simulink model "New_Model_vmaRHTS_R2019b_2"  (R2023b)
settings: Solver=ode4  StartTime=0.0  StopTime=tend  FixedStep=dt  RelTol=1e-3
values from neighbouring files (symbols this model uses):
  Ag = zeros(15,1)    [New_Full.m]
  AgN = zeros(15,1)    [New_Ns1.m]    (also in New_Ns2.m)
  AgP = zeros(6,1)    [New_Ps.m]    (also in New_Ps1.m; New_Ps2.m)
  CNrt = CRrt    [New_Ns1.m]    (also in New_Ns2.m)
  CPrt = CRrt(locate2,locate2)    [New_Ps.m]    (also in New_Ps1.m = alphas(1) * MPrt + alphas(2) * KPrt; New_Ps2.m = alphas(1) * MPrt + alphas(2) * KPrt)
  CRrt = alphas(1) * MRrt + alphas(2) * KRrt    [New_Full.m]
  dt = 1/1024    (= 0.0009765625)    [New_Full.m]
  FN = zeros(15,1)    [New_Full.m]    (also in New_Ns1.m; New_Ns2.m)
  K_P1 = zeros(6,5)    [New_Guyan.m]
  K_P2 = zeros(6,1)    [New_Guyan.m]
  Kbar_inv = inv(Kbar)    [New_Full.m]
  KNbar_inv = inv(KNbar)    [New_Ns1.m]    (also in New_Ns2.m)
  KPbar_inv = inv(KPbar)    [New_Ps.m]    (also in New_Ps1.m; New_Ps2.m)
  KPrt = KRrt(locate2,locate2)    [New_Ps.m]    (also in New_Ps1.m = [2*Kc(4,4)+2*Kc(1,1)	Kc(4,6)+Kc(1,3)	Kc(4,6)+Kc(1,3); New_Ps2.m = [2*Kc(4,4)+2*Kc(1,1)	Kc(4,6)+Kc(1,3)	Kc(4,6)+Kc(1,3)	2*Kc(1,)
  KPuc = KPrt(locate5,locate4)    [New_Guyan.m]
  KPuu = KPrt(locate5,locate5)    [New_Guyan.m]
  KRrt = [4*Kc(4,4)+4*Kc(1,1)	Kc(4,6)+Kc(1,3)	Kc(4,6)+Kc(1,3)	Kc(4,6)+Kc(1,3)	Kc(4,6)+Kc(1,3)	4*Kc(1,4)	Kc(1,6)	Kc(1,6)	Kc(1,6)	Kc(1,6)	0	0	0	0	0 ... (first row only)    [New_Full.m]
  l = zeros(15,1)    [New_Full.m]
  lN = zeros(15,1)    [New_Ns1.m]    (also in New_Ns2.m)
  locate2 = [1,2,3]    [New_Ns1.m]    (also in New_Ns2.m = [1,2,3,6,7,8]; New_Ps.m = [1,2,3,6,7,8]; New_Ps1.m = [1,2,3,6,7,8]; New_Ps2.m = [1,2,3,6,7,8])
  locate3 = zeros(15,6)    [New_Ns1.m]    (also in New_Ns2.m)
  lP = zeros(6,1)    [New_Ps.m]    (also in New_Ps1.m; New_Ps2.m)
  MNrt = diag([M5 1e-5 M6 M3 M2 M1 M2 M3 M3 M2 M1 M2 M3 M3 M2])    [New_Ns1.m]    (also in New_Ns2.m = diag([M5 1e-5 M6 M3 M2 M5 1e-5 M6 M3 M2 M1 M2 M3 M3 M2]))
  MPrt = diag([M4 M2 M3 M4 M2 M3])    [New_Ps.m]    (also in New_Ps1.m = diag([M4 M2 M2]); New_Ps2.m = diag([M4 M2 M2 M4 M2 M2]))
  MPuu = MPrt(locate5,locate5)    [New_Guyan.m]
  MRrt = diag([M1 M2 M3 M3 M2 M1 M2 M3 M3 M2 M1 M2 M3 M3 M2])    [New_Full.m]
  Rbar = zeros(15,1)    [New_Full.m]
  RNbar = zeros(15,1)    [New_Ns1.m]    (also in New_Ns2.m)
  RPbar = zeros(6,1)    [New_Ps.m]    (also in New_Ps1.m; New_Ps2.m)
  tend = 40    [New_Full.m]
undefined symbols (not defined in the file or in its folder): a0, a1, a2, a3, a4, a5, a6, a7, Ag_tilde, C_tilde, Cp_tilde, CPren, Cren, EQ_intensity, EQ_sw, F_tilde, Klocate1, KN_tilde_inv, KNren_inv, Koo, Kot, Kp_tilde, KPren, Ksmn, Ksn, l_tilde, lren, M_tilde, Mp_tilde, MPren, Mren, Phi_u0, R_tilde, Rren, T
libraries: simulink x1, sldrtlib x1
(part 1 of 2)
settings Model: Creator=icu327  LastModifiedBy=liangyu
settings DataIOCC: SaveFormat=Array  ReturnWorkspaceOutputs=off
settings DebuggingCC: UnconnectedInputMsg=warning  UnconnectedOutputMsg=warning  UnconnectedLineMsg=warning  ArithmeticOperatorsInVariantConditions=warning
settings HardwareCC: ProdBitPerLong=64  ProdHWDeviceType=Intel->x86-64 (Linux 64)
settings ModelReferenceCC: EnableRefExpFcnMdlSchedulingChecks=on
settings SFSimCC: CustomCodeUndefinedFunction=UseInterfaceOnly
settings RTWCC: Description=Simulink Desktop Real-Time  SystemTargetFile=sldrt.tlc  TemplateMakefile=sldrt.tmf  RTWCompilerOptimization=on
settings CodeAppCC: MaxIdLength=95  StateflowObjectComments=on
settings SimulinkDesktopRealTimeCC: TargetLibSuffix=_sldrt.a  TargetPreCompLibLocation=C:\Program Files\MATLAB\R2023b\toolbox\sldrt\lib\win64

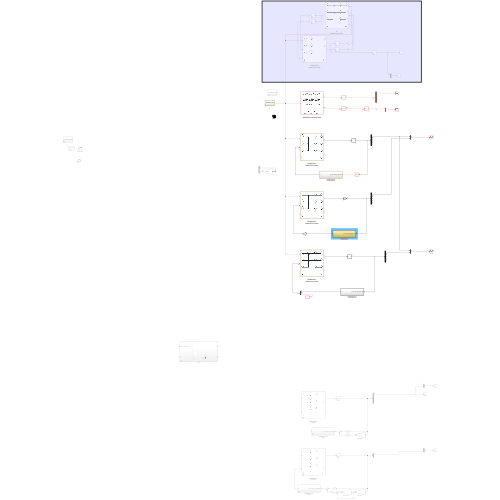
[thumbnail: Simulink's stored preview of the top-level diagram]
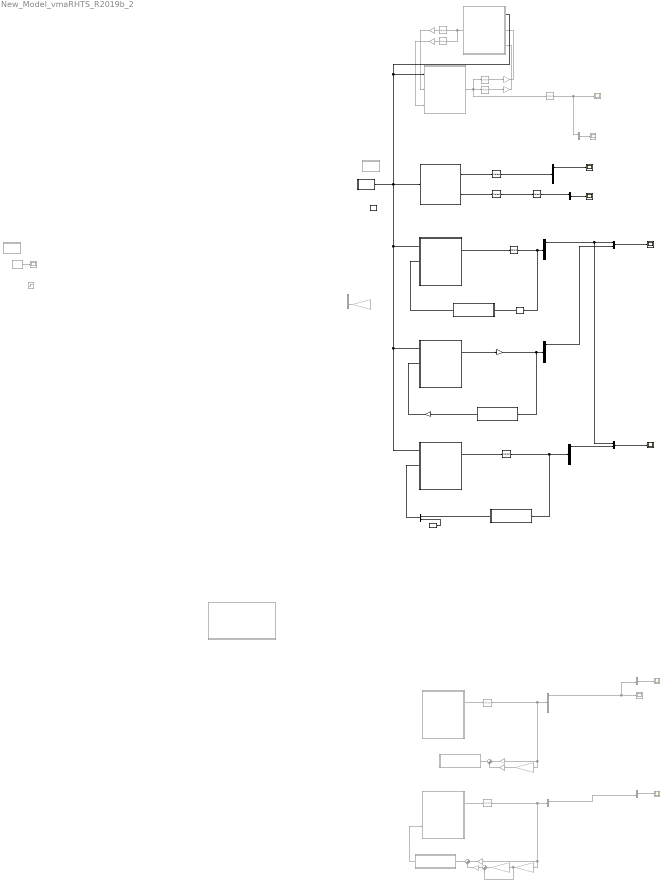
== system New_Model_vmaRHTS_R2019b_2 ==
  " 1" : Subsystem  Commented=on
  " 2" : Subsystem
  " 3" : Subsystem  Commented=on
  " NUMERICAL Guyan" : Subsystem  Commented=on
      mask Display: image('$imagefile'); % Use "Edit Image" on toolstrip to change.
  " NUMERICAL Guyan1" : Subsystem  Commented=on
      mask Display: image('$imagefile'); % Use "Edit Image" on toolstrip to change.
  " NUMERICAL SUBSTRUCTURE" : Subsystem  Commented=on
      mask Display: image('$imagefile'); % Use "Edit Image" on toolstrip to change.
  " NUMERICAL SUBSTRUCTURE1" : Subsystem
      mask Display: image('$imagefile'); % Use "Edit Image" on toolstrip to change.
  " NUMERICAL SUBSTRUCTURE2" : Subsystem
      mask Display: image('$imagefile'); % Use "Edit Image" on toolstrip to change.
  " NUMERICAL SUBSTRUCTURE3" : Subsystem
      mask Display: image('$imagefile'); % Use "Edit Image" on toolstrip to change.
  " Ps SUBSTRUCTURE1" : Subsystem  Commented=on
      mask Display: image('$imagefile'); % Use "Edit Image" on toolstrip to change.
  " REFERENCE STRUCTURE" : Subsystem
      mask Display: image('$imagefile'); % Use "Edit Image" on toolstrip to change.
  CBtest : Subsystem  Commented=on
  Chirp Signal1 : simulink/Sources/Chirp Signal  f1=0.1  T=tend  f2=10
  Constant3 : Constant  Value=zeros(3,1)  VectorParams1D=off
  Delay : Delay
  Demux : Demux  Outputs=6
  Demux1 : Demux  Outputs=6
  Demux2 : Demux  Commented=on  Outputs=5
  Demux3 : Demux  Commented=on  Outputs=2
  Demux4 : Demux  Outputs=5
  Demux5 : Demux  Outputs=5
  Feedback Force Computation1 : Subsystem
  Feedback Force Computation2 : Subsystem
  Feedback Force Computation3 : Subsystem
  Feedback Force Guyan : Subsystem  Commented=on
  Feedback Force Guyan1 : Subsystem  Commented=on
  Gain : Gain  Commented=on  Gain=K_P1  Multiplication=Matrix(K*u) (u vector)
  Gain1 : Gain  Commented=on  Gain=KRrt(3,4)  Multiplication=Matrix(K*u) (u vector)
  Gain11 : Gain  Commented=on  Gain=-inv(Koo)*Kot  Multiplication=Matrix(K*u) (u vector)
  Gain2 : Gain  Commented=on  Gain=KRrt(7:8,9:13)  Multiplication=Matrix(K*u) (u vector)
  Gain3 : Gain  Commented=on  Gain=KRrt(4,3)  Multiplication=Matrix(K*u) (u vector)
  Gain4 : Gain  Commented=on  Gain=KRrt(9:13,7:8)  Multiplication=Matrix(K*u) (u vector)
  Gain5 : Gain  Commented=on  Gain=K_P2  Multiplication=Matrix(K*u) (u vector)
  Gain6 : Gain  Commented=on  Gain=K_P1  Multiplication=Matrix(K*u) (u vector)
  Gain7 : Gain  Commented=on  Gain=K_P2  Multiplication=Matrix(K*u) (u vector)
  Gain8 : Gain  Gain=Klocate1  Multiplication=Matrix(K*u) (u vector)
  Gain9 : Gain  Gain=Klocate1'  Multiplication=Matrix(K*u) (u vector)
  Guyan增益 : Gain  Commented=on  Gain=-inv(KPuu)*KPuc  Multiplication=Matrix(K*u) (u vector)
  Guyan增益1 : Gain  Commented=on  Gain=-inv(KPuu)*KPuc  Multiplication=Matrix(K*u) (u vector)
  Guyan增益2 : Gain  Commented=on  Gain=Phi_u0*Phi_u0' * MPuu  Multiplication=Matrix(K*u) (u vector)
  Missed Ticks : Scope  Commented=on
  Mux{,6,8..9} (4 alike) : Mux  Commented=on  Inputs=2
  Mux{1..3,5} (4 alike) : Mux  Inputs=2
  Real-Time Synchronization : sldrtlib/Real-Time Synchronization  Commented=on  SampleTime=dt  MaxMissedTicks=10000  ShowMissedTicks=on  YieldWhenWaiting=off
  Scope{,3..5} (4 alike) : Scope
  Scope{1..2,11..13} (5 alike) : Scope  Commented=on
  Selector : Selector  InputPortWidth=15  IndexOptions=Index vector (dialog)  Indices=[1 2 3 6 7 8]  OutputSizes=1
  Selector1 : Selector  Commented=on  InputPortWidth=11  IndexOptions=Index vector (dialog)  Indices=[2]  OutputSizes=1
  Selector11 : Selector  InputPortWidth=6  IndexOptions=Index vector (dialog)  Indices=[1]  OutputSizes=1
  Selector12 : Selector  InputPortWidth=15  IndexOptions=Index vector (dialog)  Indices=[1 2 3 6 7 8]  OutputSizes=1
  Selector13 : Selector  Commented=on  InputPortWidth=15  IndexOptions=Index vector (dialog)  Indices=[1 3 6 7 8]  OutputSizes=1
  Selector2 : Selector  Commented=on  InputPortWidth=11  IndexOptions=Index vector (dialog)  Indices=[5 6 7 8 9]  OutputSizes=1
  Selector3 : Selector  Commented=on  InputPortWidth=15  IndexOptions=Index vector (dialog)  Indices=[1 3 6 7 8]  OutputSizes=1
  Selector4 : Selector  Commented=on  InputPortWidth=11  IndexOptions=Index vector (dialog)  Indices=[1]  OutputSizes=1
  Selector5 : Selector  InputPortWidth=15  IndexOptions=Index vector (dialog)  Indices=[1 2 3 6 7 8]  OutputSizes=1
  Selector6 : Selector  Commented=on  InputPortWidth=6  IndexOptions=Index vector (dialog)  Indices=[3]  OutputSizes=1
  Selector7 : Selector  Commented=on  InputPortWidth=6  IndexOptions=Index vector (dialog)  Indices=[5 6]  OutputSizes=1
  Selector8 : Selector  InputPortWidth=8  IndexOptions=Index vector (dialog)  Indices=[1 2 3 4 5]  OutputSizes=1
  Step5 : Step  Commented=on  SampleTime=0
  Sum : Sum  Commented=on  Inputs=|++
  Sum2 : Sum  Commented=on  Inputs=|++
  Sum3 : Sum  Commented=on  Inputs=|++
  wires:
  Real-Time Synchronization/1 -> Missed Ticks/1
  " REFERENCE STRUCTURE"/1(Output) -> Selector5/1
  Mux/1 -> Scope2/1
  " Ps SUBSTRUCTURE1"/1(Output) -> Selector7/1, Selector6/1
  Selector4/1 -> Scope1/1, Mux/1
  Selector2/1 -> Gain2/1
  Selector1/1 -> Gain1/1
  Gain1/1 -> " Ps SUBSTRUCTURE1"/2(Input)
  Gain2/1 -> " Ps SUBSTRUCTURE1"/3(Input1)
  Selector6/1 -> Gain3/1
  Gain3/1 -> " NUMERICAL SUBSTRUCTURE"/2(Input)
  Selector7/1 -> Gain4/1
  Gain4/1 -> " NUMERICAL SUBSTRUCTURE"/3(Input1)
  " NUMERICAL SUBSTRUCTURE"/1(Output) -> Selector4/1, Selector1/1, Selector2/1
  Selector12/1 -> Selector11/1
  " REFERENCE STRUCTURE"/2(Output1) -> Selector12/1
  Selector11/1 -> Mux1/1  "Rs"
  Mux1/1 -> Scope3/1
  Selector5/1 -> Demux1/1  "Rs"
  Demux1/1 -> Scope4/1
  " NUMERICAL Guyan"/1(Output) -> Selector3/1
  Guyan增益/1 -> Gain5/1
  Sum/1 -> Feedback Force Guyan/1("[x_est, theta_est] (m,rad)")
  Gain/1 -> Sum/1
  Gain5/1 -> Sum/2
  Demux2/1 -> Scope11/1, Mux8/2  "Ns"
  Mux8/1 -> Scope12/1
  Gain6/1 -> Sum2/1
  Feedback Force Guyan1/1(Output) -> " NUMERICAL Guyan1"/2(Input)
  Guyan增益1/1 -> Guyan增益2/1, Sum3/2
  Sum2/1 -> Feedback Force Guyan1/1("[x_est, theta_est] (m,rad)")
  " NUMERICAL Guyan1"/1(Output) -> Selector13/1
  Gain7/1 -> Sum2/2
  Guyan增益2/1 -> Sum3/1
  Sum3/1 -> Gain7/1
  Demux3/1 -> Mux9/2  "Ns"
  Mux9/1 -> Scope13/1
  Selector3/1 -> Demux2/1, Guyan增益/1, Gain/1
  Selector13/1 -> Demux3/1, Guyan增益1/1, Gain6/1
  Feedback Force Computation3/1(Output) -> " NUMERICAL SUBSTRUCTURE1"/2(Input)
  Gain9/1 -> " NUMERICAL SUBSTRUCTURE2"/2(Input)
  Demux4/1 -> Mux2/2  "Ns"
  ? -> Gain11/1
  ? -> Mux6/1
  Gain11/1 -> Mux6/2
  Gain8/1 -> Feedback Force Computation1/1("[x_est, theta_est] (m,rad)"), Demux4/1
  " NUMERICAL SUBSTRUCTURE3"/1(Output) -> Selector8/1
  " 2"/1(GROUND ACCEL) -> " NUMERICAL SUBSTRUCTURE2"/1(Ground_Acceleration), " NUMERICAL SUBSTRUCTURE3"/1(Ground_Acceleration), " NUMERICAL SUBSTRUCTURE1"/1(Ground_Acceleration), " NUMERICAL SUBSTRUCTURE"/1(Ground_Acceleration), " Ps SUBSTRUCTURE1"/1(Ground_Acceleration), " REFERENCE STRUCTURE"/1(Ground_Acceleration)
  Mux5/1 -> " NUMERICAL SUBSTRUCTURE3"/2(Input)
  Constant3/1 -> Mux5/2
  Selector8/1 -> Feedback Force Computation2/1("[x_est, theta_est] (m,rad)"), Demux5/1
  Feedback Force Computation2/1(Output) -> Mux5/1
  Feedback Force Computation1/1(Output) -> Gain9/1
  " NUMERICAL SUBSTRUCTURE2"/1(Output) -> Gain8/1
  " NUMERICAL SUBSTRUCTURE1"/1(Output) -> Selector/1
  Demux/1 -> Mux3/1, Mux2/1  "Ns"
  Mux2/1 -> Scope/1
  Mux3/1 -> Scope5/1
  Demux5/1 -> Mux3/2  "Ns"
  Selector/1 -> Delay/1, Demux/1
  Delay/1 -> Feedback Force Computation3/1("[x_est, theta_est] (m,rad)")

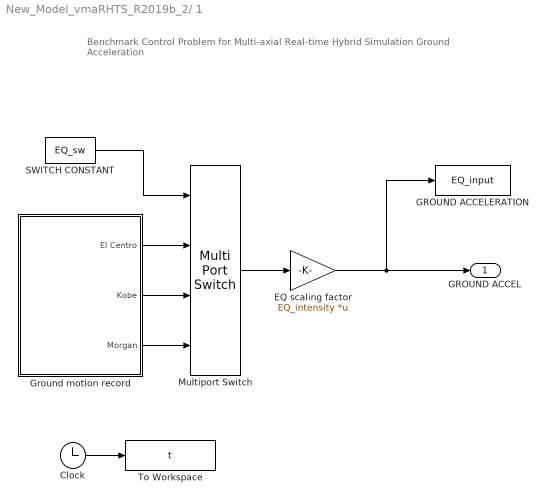
== system New_Model_vmaRHTS_R2019b_2/ 1 ==
  note: Benchmark Control Problem for
      | Multi-axial Real-time Hybrid Simulation
      | Ground Acceleration
  Clock : Clock
  EQ scaling factor : Gain  Gain=EQ_intensity  Multiplication=Matrix(K*u)
  GROUND ACCELERATION : ToWorkspace  VariableName=EQ_input  SampleTime=-1
      settings: Save2DSignal=2-D array (concatenate along first dimension)
  Ground motion record : Subsystem
  Multiport Switch : MultiPortSwitch  SaturateOnIntegerOverflow=off  InputSameDT=off
  SWITCH CONSTANT : Constant  Value=EQ_sw
  To Workspace : ToWorkspace  VariableName=t  SampleTime=dt
  GROUND ACCEL : Outport  VectorParamsAs1DForOutWhenUnconnected=off
  wires:
  Multiport Switch/1 -> EQ scaling factor/1
  EQ scaling factor/1 -> GROUND ACCELERATION/1, GROUND ACCEL/1
  Ground motion record/1(El Centro) -> Multiport Switch/2
  Ground motion record/2(Kobe) -> Multiport Switch/3
  Ground motion record/3(Morgan) -> Multiport Switch/4
  SWITCH CONSTANT/1 -> Multiport Switch/1
  Clock/1 -> To Workspace/1

== system New_Model_vmaRHTS_R2019b_2/ 2 ==
  note: Benchmark Control Problem for
      | Multi-axial Real-time Hybrid Simulation
      | Ground Acceleration
  Clock : Clock
  EQ scaling factor : Gain  Gain=EQ_intensity  Multiplication=Matrix(K*u)
  GROUND ACCELERATION : ToWorkspace  VariableName=EQ_input  SampleTime=-1
      settings: Save2DSignal=2-D array (concatenate along first dimension)
  Ground motion record : Subsystem
  Multiport Switch : MultiPortSwitch  SaturateOnIntegerOverflow=off  InputSameDT=off
  SWITCH CONSTANT : Constant  Value=EQ_sw
  To Workspace : ToWorkspace  VariableName=t  SampleTime=dt
  GROUND ACCEL : Outport  VectorParamsAs1DForOutWhenUnconnected=off
  wires:
  Multiport Switch/1 -> EQ scaling factor/1
  EQ scaling factor/1 -> GROUND ACCELERATION/1, GROUND ACCEL/1
  Ground motion record/1(El Centro) -> Multiport Switch/2
  Ground motion record/2(Kobe) -> Multiport Switch/3
  Ground motion record/3(Morgan) -> Multiport Switch/4
  SWITCH CONSTANT/1 -> Multiport Switch/1
  Clock/1 -> To Workspace/1

== system New_Model_vmaRHTS_R2019b_2/ 3 ==
  note: Benchmark Control Problem for
      | Multi-axial Real-time Hybrid Simulation
      | Ground Acceleration
  Clock : Clock
  EQ scaling factor : Gain  Gain=EQ_intensity  Multiplication=Matrix(K*u)
  GROUND ACCELERATION : ToWorkspace  VariableName=EQ_input  SampleTime=-1
      settings: Save2DSignal=2-D array (concatenate along first dimension)
  Ground motion record : Subsystem
  Multiport Switch : MultiPortSwitch  SaturateOnIntegerOverflow=off  InputSameDT=off
  SWITCH CONSTANT : Constant  Value=EQ_sw
  To Workspace : ToWorkspace  VariableName=t  SampleTime=dt
  GROUND ACCEL : Outport  VectorParamsAs1DForOutWhenUnconnected=off
  wires:
  Multiport Switch/1 -> EQ scaling factor/1
  EQ scaling factor/1 -> GROUND ACCELERATION/1, GROUND ACCEL/1
  Ground motion record/1(El Centro) -> Multiport Switch/2
  Ground motion record/2(Kobe) -> Multiport Switch/3
  Ground motion record/3(Morgan) -> Multiport Switch/4
  SWITCH CONSTANT/1 -> Multiport Switch/1
  Clock/1 -> To Workspace/1

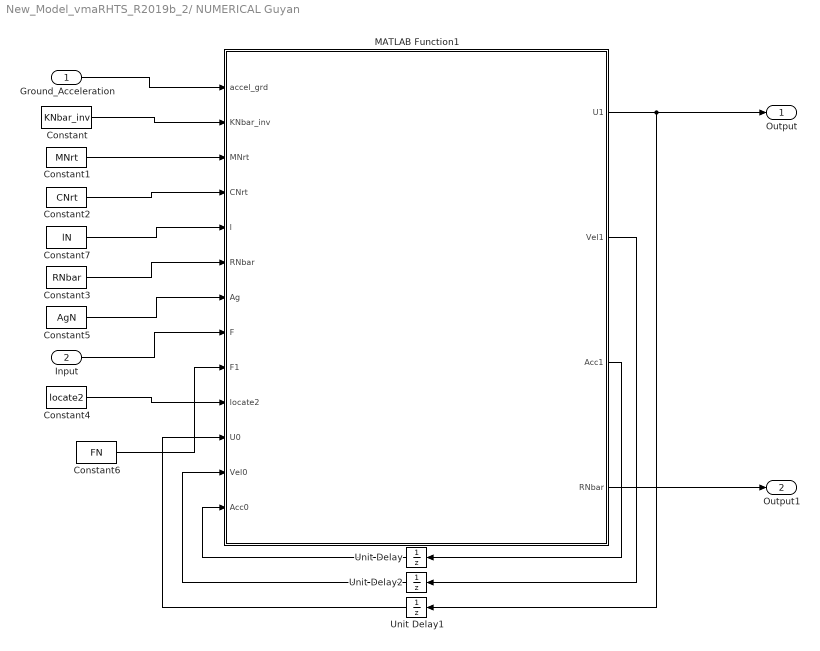
== system New_Model_vmaRHTS_R2019b_2/ NUMERICAL Guyan ==
  Ground_Acceleration : Inport
  Input : Inport  Port=2
  Constant : Constant  Value=KNbar_inv  VectorParams1D=off
  Constant1 : Constant  Value=MNrt  VectorParams1D=off
  Constant2 : Constant  Value=CNrt  VectorParams1D=off
  Constant3 : Constant  Value=RNbar  VectorParams1D=off
  Constant4 : Constant  Value=locate2  VectorParams1D=off
  Constant5 : Constant  Value=AgN  VectorParams1D=off
  Constant6 : Constant  Value=FN  VectorParams1D=off
  Constant7 : Constant  Value=lN  VectorParams1D=off
  MATLAB Function1 : MATLAB Function  TreatAsAtomicUnit=on
  Unit Delay : UnitDelay  SampleTime=-1  HasFrameUpgradeWarning=on
  Unit Delay1 : UnitDelay  SampleTime=-1  HasFrameUpgradeWarning=on
  Unit Delay2 : UnitDelay  SampleTime=-1  HasFrameUpgradeWarning=on
  Output : Outport
  Output1 : Outport  Port=2
  wires:
  Ground_Acceleration/1 -> MATLAB Function1/1(accel_grd)
  Constant/1 -> MATLAB Function1/2(KNbar_inv)
  Constant1/1 -> MATLAB Function1/3(MNrt)
  Constant2/1 -> MATLAB Function1/4(CNrt)
  Constant7/1 -> MATLAB Function1/5(l)
  Unit Delay2/1 -> MATLAB Function1/12(Vel0)
  Unit Delay/1 -> MATLAB Function1/13(Acc0)
  MATLAB Function1/2(Vel1) -> Unit Delay2/1
  MATLAB Function1/3(Acc1) -> Unit Delay/1
  Constant5/1 -> MATLAB Function1/7(Ag)
  Unit Delay1/1 -> MATLAB Function1/11(U0)
  Constant3/1 -> MATLAB Function1/6("RNbar ")
  Input/1 -> MATLAB Function1/8(F)
  MATLAB Function1/1(U1) -> Output/1, Unit Delay1/1
  Constant4/1 -> MATLAB Function1/10(locate2)
  Constant6/1 -> MATLAB Function1/9(F1)
  MATLAB Function1/4(RNbar) -> Output1/1

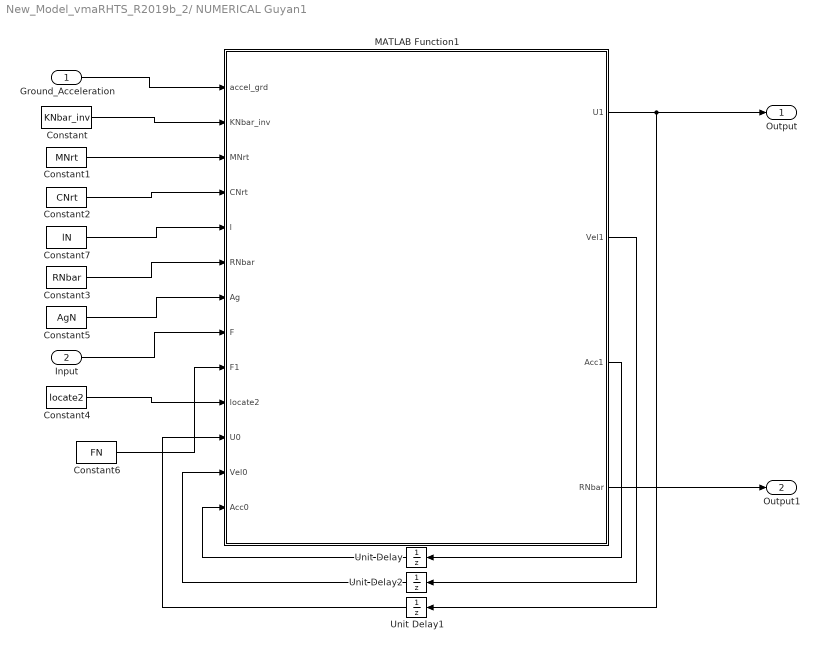
== system New_Model_vmaRHTS_R2019b_2/ NUMERICAL Guyan1 ==
  Ground_Acceleration : Inport
  Input : Inport  Port=2
  Constant : Constant  Value=KNbar_inv  VectorParams1D=off
  Constant1 : Constant  Value=MNrt  VectorParams1D=off
  Constant2 : Constant  Value=CNrt  VectorParams1D=off
  Constant3 : Constant  Value=RNbar  VectorParams1D=off
  Constant4 : Constant  Value=locate2  VectorParams1D=off
  Constant5 : Constant  Value=AgN  VectorParams1D=off
  Constant6 : Constant  Value=FN  VectorParams1D=off
  Constant7 : Constant  Value=lN  VectorParams1D=off
  MATLAB Function1 : MATLAB Function  TreatAsAtomicUnit=on
  Unit Delay : UnitDelay  SampleTime=-1  HasFrameUpgradeWarning=on
  Unit Delay1 : UnitDelay  SampleTime=-1  HasFrameUpgradeWarning=on
  Unit Delay2 : UnitDelay  SampleTime=-1  HasFrameUpgradeWarning=on
  Output : Outport
  Output1 : Outport  Port=2
  wires:
  Ground_Acceleration/1 -> MATLAB Function1/1(accel_grd)
  Constant/1 -> MATLAB Function1/2(KNbar_inv)
  Constant1/1 -> MATLAB Function1/3(MNrt)
  Constant2/1 -> MATLAB Function1/4(CNrt)
  Constant7/1 -> MATLAB Function1/5(l)
  Unit Delay2/1 -> MATLAB Function1/12(Vel0)
  Unit Delay/1 -> MATLAB Function1/13(Acc0)
  MATLAB Function1/2(Vel1) -> Unit Delay2/1
  MATLAB Function1/3(Acc1) -> Unit Delay/1
  Constant5/1 -> MATLAB Function1/7(Ag)
  Unit Delay1/1 -> MATLAB Function1/11(U0)
  Constant3/1 -> MATLAB Function1/6("RNbar ")
  Input/1 -> MATLAB Function1/8(F)
  MATLAB Function1/1(U1) -> Output/1, Unit Delay1/1
  Constant4/1 -> MATLAB Function1/10(locate2)
  Constant6/1 -> MATLAB Function1/9(F1)
  MATLAB Function1/4(RNbar) -> Output1/1

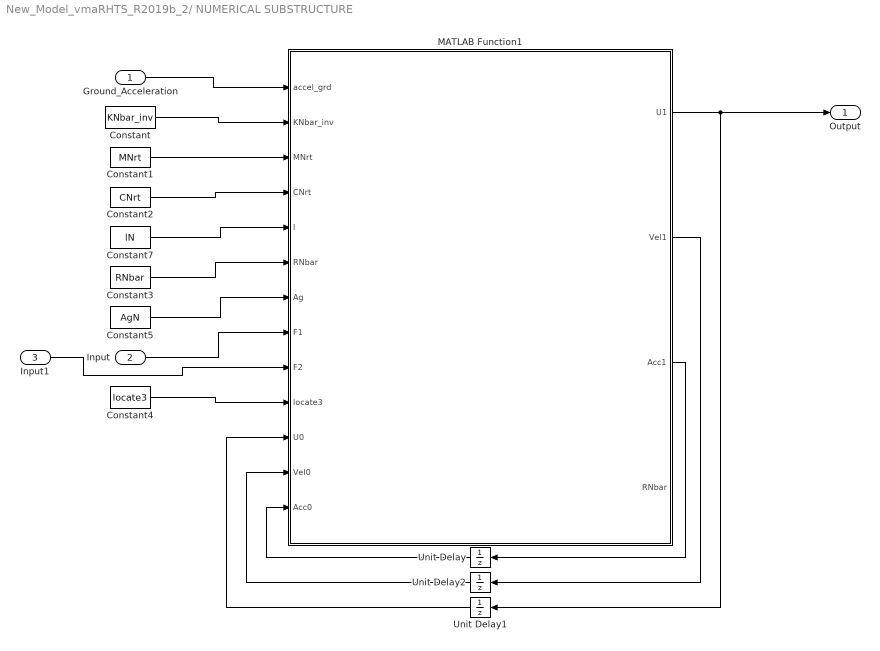
== system New_Model_vmaRHTS_R2019b_2/ NUMERICAL SUBSTRUCTURE ==
  Ground_Acceleration : Inport
  Input : Inport  Port=2
  Input1 : Inport  Port=3
  Constant : Constant  Value=KNbar_inv  VectorParams1D=off
  Constant1 : Constant  Value=MNrt  VectorParams1D=off
  Constant2 : Constant  Value=CNrt  VectorParams1D=off
  Constant3 : Constant  Value=RNbar  VectorParams1D=off
  Constant4 : Constant  Value=locate3  VectorParams1D=off
  Constant5 : Constant  Value=AgN  VectorParams1D=off
  Constant7 : Constant  Value=lN  VectorParams1D=off
  MATLAB Function1 : MATLAB Function  TreatAsAtomicUnit=on
  Unit Delay : UnitDelay  SampleTime=-1  HasFrameUpgradeWarning=on
  Unit Delay1 : UnitDelay  SampleTime=-1  HasFrameUpgradeWarning=on
  Unit Delay2 : UnitDelay  SampleTime=-1  HasFrameUpgradeWarning=on
  Output : Outport
  wires:
  Ground_Acceleration/1 -> MATLAB Function1/1(accel_grd)
  Constant/1 -> MATLAB Function1/2(KNbar_inv)
  Constant1/1 -> MATLAB Function1/3(MNrt)
  Constant2/1 -> MATLAB Function1/4(CNrt)
  Constant7/1 -> MATLAB Function1/5(l)
  Unit Delay2/1 -> MATLAB Function1/12(Vel0)
  Unit Delay/1 -> MATLAB Function1/13(Acc0)
  MATLAB Function1/2(Vel1) -> Unit Delay2/1
  MATLAB Function1/3(Acc1) -> Unit Delay/1
  Constant5/1 -> MATLAB Function1/7(Ag)
  Unit Delay1/1 -> MATLAB Function1/11(U0)
  Constant3/1 -> MATLAB Function1/6("RNbar ")
  Input/1 -> MATLAB Function1/8(F1)
  MATLAB Function1/1(U1) -> Output/1, Unit Delay1/1
  Constant4/1 -> MATLAB Function1/10(locate3)
  Input1/1 -> MATLAB Function1/9(F2)

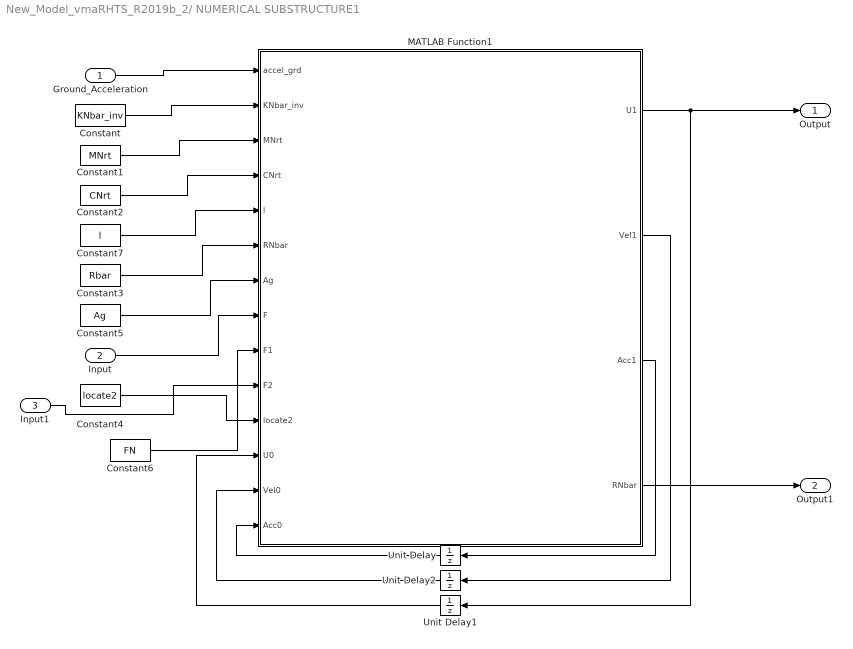
== system New_Model_vmaRHTS_R2019b_2/ NUMERICAL SUBSTRUCTURE1 ==
  Ground_Acceleration : Inport
  Input : Inport  Port=2
  Input1 : Inport  Port=3
  Constant : Constant  Value=KNbar_inv  VectorParams1D=off
  Constant1 : Constant  Value=MNrt  VectorParams1D=off
  Constant2 : Constant  Value=CNrt  VectorParams1D=off
  Constant3 : Constant  Value=Rbar  VectorParams1D=off
  Constant4 : Constant  Value=locate2  VectorParams1D=off
  Constant5 : Constant  Value=Ag  VectorParams1D=off
  Constant6 : Constant  Value=FN  VectorParams1D=off
  Constant7 : Constant  Value=l  VectorParams1D=off
  MATLAB Function1 : MATLAB Function  TreatAsAtomicUnit=on
  Unit Delay : UnitDelay  SampleTime=-1  HasFrameUpgradeWarning=on
  Unit Delay1 : UnitDelay  SampleTime=-1  HasFrameUpgradeWarning=on
  Unit Delay2 : UnitDelay  SampleTime=-1  HasFrameUpgradeWarning=on
  Output : Outport
  Output1 : Outport  Port=2
  wires:
  Ground_Acceleration/1 -> MATLAB Function1/1(accel_grd)
  Constant/1 -> MATLAB Function1/2(KNbar_inv)
  Constant1/1 -> MATLAB Function1/3(MNrt)
  Constant2/1 -> MATLAB Function1/4(CNrt)
  Constant7/1 -> MATLAB Function1/5(l)
  Unit Delay2/1 -> MATLAB Function1/13(Vel0)
  Unit Delay/1 -> MATLAB Function1/14(Acc0)
  MATLAB Function1/2(Vel1) -> Unit Delay2/1
  MATLAB Function1/3(Acc1) -> Unit Delay/1
  Constant5/1 -> MATLAB Function1/7(Ag)
  Unit Delay1/1 -> MATLAB Function1/12(U0)
  Constant3/1 -> MATLAB Function1/6("RNbar ")
  Input/1 -> MATLAB Function1/8(F)
  MATLAB Function1/1(U1) -> Output/1, Unit Delay1/1
  Constant4/1 -> MATLAB Function1/11(locate2)
  Constant6/1 -> MATLAB Function1/9(F1)
  MATLAB Function1/4(RNbar) -> Output1/1
  Input1/1 -> MATLAB Function1/10(F2)

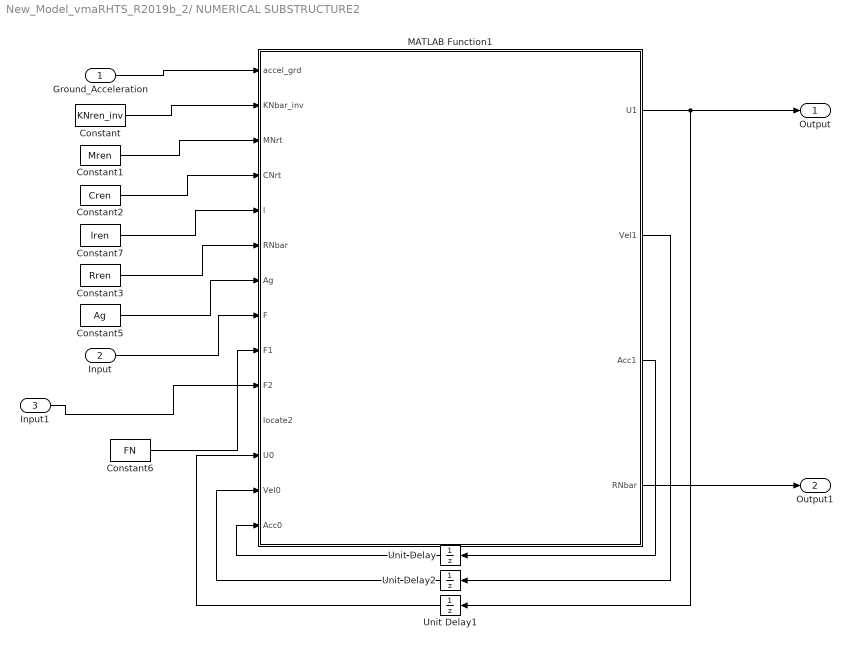
== system New_Model_vmaRHTS_R2019b_2/ NUMERICAL SUBSTRUCTURE2 ==
  Ground_Acceleration : Inport
  Input : Inport  Port=2
  Input1 : Inport  Port=3
  Constant : Constant  Value=KNren_inv  VectorParams1D=off
  Constant1 : Constant  Value=Mren  VectorParams1D=off
  Constant2 : Constant  Value=Cren  VectorParams1D=off
  Constant3 : Constant  Value=Rren  VectorParams1D=off
  Constant5 : Constant  Value=Ag  VectorParams1D=off
  Constant6 : Constant  Value=FN  VectorParams1D=off
  Constant7 : Constant  Value=lren  VectorParams1D=off
  MATLAB Function1 : MATLAB Function  TreatAsAtomicUnit=on
  Unit Delay : UnitDelay  SampleTime=-1  HasFrameUpgradeWarning=on
  Unit Delay1 : UnitDelay  SampleTime=-1  HasFrameUpgradeWarning=on
  Unit Delay2 : UnitDelay  SampleTime=-1  HasFrameUpgradeWarning=on
  Output : Outport
  Output1 : Outport  Port=2
  wires:
  Ground_Acceleration/1 -> MATLAB Function1/1(accel_grd)
  Constant/1 -> MATLAB Function1/2(KNbar_inv)
  Constant1/1 -> MATLAB Function1/3(MNrt)
  Constant2/1 -> MATLAB Function1/4(CNrt)
  Constant7/1 -> MATLAB Function1/5(l)
  Unit Delay2/1 -> MATLAB Function1/13(Vel0)
  Unit Delay/1 -> MATLAB Function1/14(Acc0)
  MATLAB Function1/2(Vel1) -> Unit Delay2/1
  MATLAB Function1/3(Acc1) -> Unit Delay/1
  Constant5/1 -> MATLAB Function1/7(Ag)
  Unit Delay1/1 -> MATLAB Function1/12(U0)
  Constant3/1 -> MATLAB Function1/6("RNbar ")
  Input/1 -> MATLAB Function1/8(F)
  MATLAB Function1/1(U1) -> Output/1, Unit Delay1/1
  Constant6/1 -> MATLAB Function1/9(F1)
  MATLAB Function1/4(RNbar) -> Output1/1
  Input1/1 -> MATLAB Function1/10(F2)

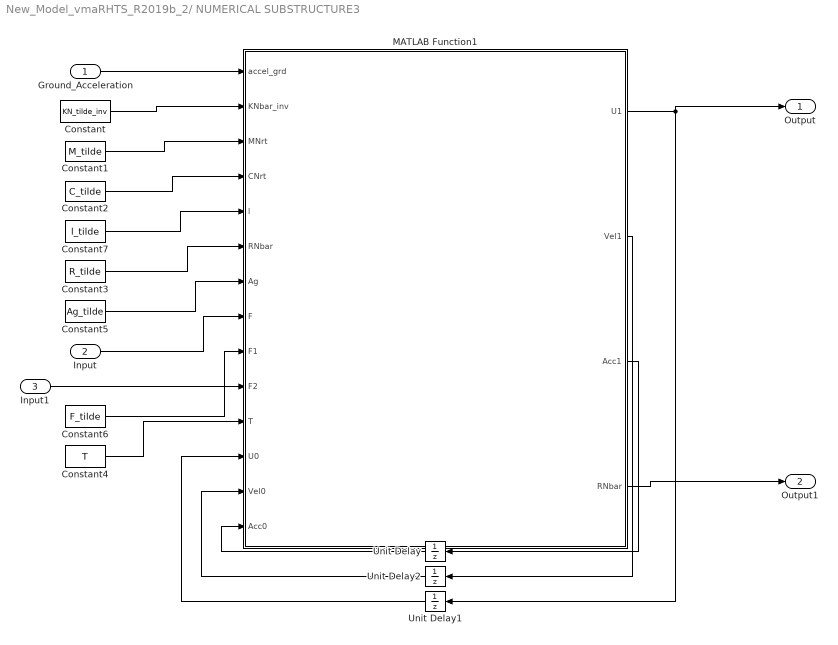
== system New_Model_vmaRHTS_R2019b_2/ NUMERICAL SUBSTRUCTURE3 ==
  Ground_Acceleration : Inport
  Input : Inport  Port=2
  Input1 : Inport  Port=3
  Constant : Constant  Value=KN_tilde_inv  VectorParams1D=off
  Constant1 : Constant  Value=M_tilde  VectorParams1D=off
  Constant2 : Constant  Value=C_tilde  VectorParams1D=off
  Constant3 : Constant  Value=R_tilde  VectorParams1D=off
  Constant4 : Constant  Value=T  VectorParams1D=off
  Constant5 : Constant  Value=Ag_tilde  VectorParams1D=off
  Constant6 : Constant  Value=F_tilde  VectorParams1D=off
  Constant7 : Constant  Value=l_tilde  VectorParams1D=off
  MATLAB Function1 : MATLAB Function  TreatAsAtomicUnit=on
  Unit Delay : UnitDelay  SampleTime=-1  HasFrameUpgradeWarning=on
  Unit Delay1 : UnitDelay  SampleTime=-1  HasFrameUpgradeWarning=on
  Unit Delay2 : UnitDelay  SampleTime=-1  HasFrameUpgradeWarning=on
  Output : Outport
  Output1 : Outport  Port=2
  wires:
  Ground_Acceleration/1 -> MATLAB Function1/1(accel_grd)
  Constant/1 -> MATLAB Function1/2(KNbar_inv)
  Constant1/1 -> MATLAB Function1/3(MNrt)
  Constant2/1 -> MATLAB Function1/4(CNrt)
  Constant7/1 -> MATLAB Function1/5(l)
  Unit Delay2/1 -> MATLAB Function1/13(Vel0)
  Unit Delay/1 -> MATLAB Function1/14(Acc0)
  MATLAB Function1/2(Vel1) -> Unit Delay2/1
  MATLAB Function1/3(Acc1) -> Unit Delay/1
  Constant5/1 -> MATLAB Function1/7(Ag)
  Unit Delay1/1 -> MATLAB Function1/12(U0)
  Constant3/1 -> MATLAB Function1/6("RNbar ")
  Input/1 -> MATLAB Function1/8(F)
  MATLAB Function1/1(U1) -> Output/1, Unit Delay1/1
  Constant6/1 -> MATLAB Function1/9(F1)
  MATLAB Function1/4(RNbar) -> Output1/1
  Input1/1 -> MATLAB Function1/10(F2)
  Constant4/1 -> MATLAB Function1/11(T)

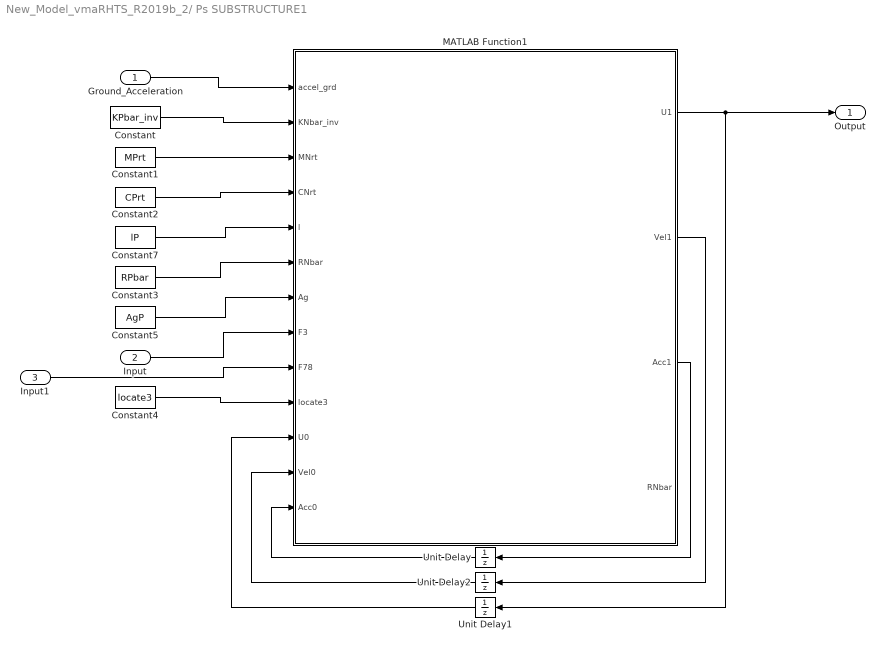
== system New_Model_vmaRHTS_R2019b_2/ Ps SUBSTRUCTURE1 ==
  Ground_Acceleration : Inport
  Input : Inport  Port=2
  Input1 : Inport  Port=3
  Constant : Constant  Value=KPbar_inv  VectorParams1D=off
  Constant1 : Constant  Value=MPrt  VectorParams1D=off
  Constant2 : Constant  Value=CPrt  VectorParams1D=off
  Constant3 : Constant  Value=RPbar  VectorParams1D=off
  Constant4 : Constant  Value=locate3  VectorParams1D=off
  Constant5 : Constant  Value=AgP  VectorParams1D=off
  Constant7 : Constant  Value=lP  VectorParams1D=off
  MATLAB Function1 : MATLAB Function  TreatAsAtomicUnit=on
  Unit Delay : UnitDelay  SampleTime=-1  HasFrameUpgradeWarning=on
  Unit Delay1 : UnitDelay  SampleTime=-1  HasFrameUpgradeWarning=on
  Unit Delay2 : UnitDelay  SampleTime=-1  HasFrameUpgradeWarning=on
  Output : Outport
  wires:
  Ground_Acceleration/1 -> MATLAB Function1/1(accel_grd)
  Constant/1 -> MATLAB Function1/2(KNbar_inv)
  Constant1/1 -> MATLAB Function1/3(MNrt)
  Constant2/1 -> MATLAB Function1/4(CNrt)
  Constant7/1 -> MATLAB Function1/5(l)
  Unit Delay2/1 -> MATLAB Function1/12(Vel0)
  Unit Delay/1 -> MATLAB Function1/13(Acc0)
  MATLAB Function1/2(Vel1) -> Unit Delay2/1
  MATLAB Function1/3(Acc1) -> Unit Delay/1
  Constant5/1 -> MATLAB Function1/7(Ag)
  Unit Delay1/1 -> MATLAB Function1/11(U0)
  Constant3/1 -> MATLAB Function1/6("RNbar ")
  Input/1 -> MATLAB Function1/8(F3)
  MATLAB Function1/1(U1) -> Output/1, Unit Delay1/1
  Constant4/1 -> MATLAB Function1/10(locate3)
  Input1/1 -> MATLAB Function1/9(F78)

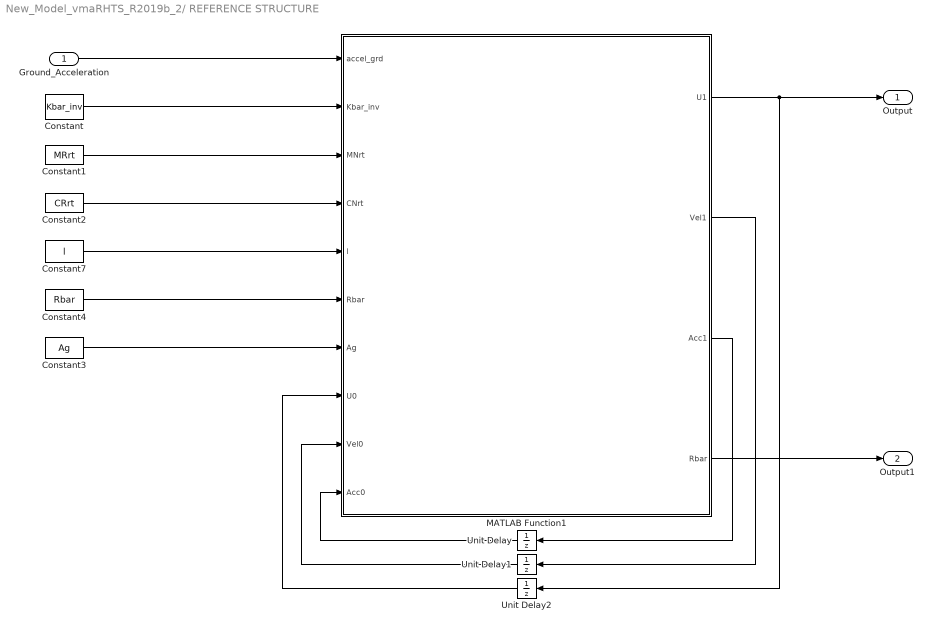
== system New_Model_vmaRHTS_R2019b_2/ REFERENCE STRUCTURE ==
  Ground_Acceleration : Inport
  Constant : Constant  Value=Kbar_inv  VectorParams1D=off
  Constant1 : Constant  Value=MRrt  VectorParams1D=off
  Constant2 : Constant  Value=CRrt  VectorParams1D=off
  Constant3 : Constant  Value=Ag  VectorParams1D=off
  Constant4 : Constant  Value=Rbar  VectorParams1D=off
  Constant7 : Constant  Value=l  VectorParams1D=off
  MATLAB Function1 : MATLAB Function  TreatAsAtomicUnit=on
  Unit Delay : UnitDelay  SampleTime=-1  HasFrameUpgradeWarning=on
  Unit Delay1 : UnitDelay  SampleTime=-1  HasFrameUpgradeWarning=on
  Unit Delay2 : UnitDelay  SampleTime=-1  HasFrameUpgradeWarning=on
  Output : Outport
  Output1 : Outport  Port=2
  wires:
  Ground_Acceleration/1 -> MATLAB Function1/1(accel_grd)
  Constant/1 -> MATLAB Function1/2(Kbar_inv)
  Constant1/1 -> MATLAB Function1/3(MNrt)
  Constant2/1 -> MATLAB Function1/4(CNrt)
  Constant7/1 -> MATLAB Function1/5(l)
  Constant4/1 -> MATLAB Function1/6("Rbar ")
  Unit Delay2/1 -> MATLAB Function1/8(U0)
  Unit Delay1/1 -> MATLAB Function1/9(Vel0)
  Unit Delay/1 -> MATLAB Function1/10(Acc0)
  MATLAB Function1/2(Vel1) -> Unit Delay1/1
  MATLAB Function1/3(Acc1) -> Unit Delay/1
  MATLAB Function1/1(U1) -> Output/1, Unit Delay2/1
  MATLAB Function1/4(Rbar) -> Output1/1
  Constant3/1 -> MATLAB Function1/7(Ag)

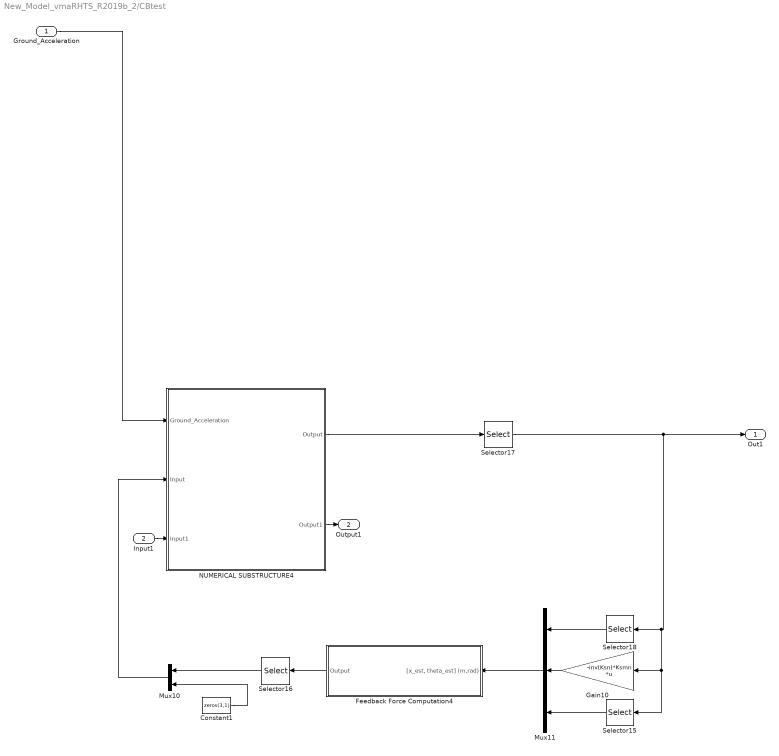
== system New_Model_vmaRHTS_R2019b_2/CBtest ==
  Ground_Acceleration : Inport
  Input1 : Inport  Port=2
  " NUMERICAL SUBSTRUCTURE4" : Subsystem
      mask Display: image('$imagefile'); % Use "Edit Image" on toolstrip to change.
  Constant1 : Constant  Value=zeros(3,1)  VectorParams1D=off
  Feedback Force Computation4 : Subsystem
  Gain10 : Gain  Gain=-inv(Ksn)*Ksmn  Multiplication=Matrix(K*u) (u vector)
  Mux10 : Mux  Inputs=2
  Mux11 : Mux  Inputs=3
  Selector15 : Selector  InputPortWidth=5  IndexOptions=Index vector (dialog)  Indices=[2 3 4 5]  OutputSizes=1
  Selector16 : Selector  InputPortWidth=6  IndexOptions=Index vector (dialog)  Indices=[1 2 3 4 5]  OutputSizes=1
  Selector17 : Selector  InputPortWidth=8  IndexOptions=Index vector (dialog)  Indices=[1 2 3 4 5]  OutputSizes=1
  Selector18 : Selector  InputPortWidth=5  IndexOptions=Index vector (dialog)  Indices=[1]  OutputSizes=1
  Out1 : Outport
  Output1 : Outport  Port=2
  wires:
  Selector15/1 -> Mux11/3
  Mux11/1 -> Feedback Force Computation4/1("[x_est, theta_est] (m,rad)")
  " NUMERICAL SUBSTRUCTURE4"/1(Output) -> Selector17/1
  Feedback Force Computation4/1(Output) -> Selector16/1
  Constant1/1 -> Mux10/2
  Mux10/1 -> " NUMERICAL SUBSTRUCTURE4"/2(Input)
  Selector16/1 -> Mux10/1
  Gain10/1 -> Mux11/2
  Selector17/1 -> Out1/1, Selector18/1, Selector15/1, Gain10/1
  Selector18/1 -> Mux11/1
  Ground_Acceleration/1 -> " NUMERICAL SUBSTRUCTURE4"/1(Ground_Acceleration)
  Input1/1 -> " NUMERICAL SUBSTRUCTURE4"/3(Input1)
  " NUMERICAL SUBSTRUCTURE4"/2(Output1) -> Output1/1

== system New_Model_vmaRHTS_R2019b_2/Feedback Force Computation1 ==
  "[x_est, theta_est] (m,rad)" : Inport
  Derivative : Derivative
  Derivative1 : Derivative
  Gain1 : Gain  Gain=KPren  Multiplication=Matrix(K*u) (u vector)
  Gain2 : Gain  Gain=CPren  Multiplication=Matrix(K*u) (u vector)
  Gain3 : Gain  Gain=MPren  Multiplication=Matrix(K*u) (u vector)
  Sum : Sum  Inputs=+|+|+
  Output : Outport
  wires:
  Derivative1/1 -> Gain3/1
  Gain2/1 -> Sum/2
  Derivative/1 -> Gain2/1, Derivative1/1
  Gain1/1 -> Sum/1
  Sum/1 -> Output/1
  Gain3/1 -> Sum/3
  "[x_est, theta_est] (m,rad)"/1 -> Derivative/1, Gain1/1

== system New_Model_vmaRHTS_R2019b_2/Feedback Force Computation2 ==
  "[x_est, theta_est] (m,rad)" : Inport
  Derivative : Derivative
  Derivative1 : Derivative
  Gain1 : Gain  Gain=KPren  Multiplication=Matrix(K*u) (u vector)
  Gain2 : Gain  Gain=CPren  Multiplication=Matrix(K*u) (u vector)
  Gain3 : Gain  Gain=MPren  Multiplication=Matrix(K*u) (u vector)
  Sum : Sum  Inputs=+|+|+
  Output : Outport
  wires:
  Derivative1/1 -> Gain3/1
  Gain2/1 -> Sum/2
  Derivative/1 -> Gain2/1, Derivative1/1
  Gain1/1 -> Sum/1
  Sum/1 -> Output/1
  Gain3/1 -> Sum/3
  "[x_est, theta_est] (m,rad)"/1 -> Derivative/1, Gain1/1

== system New_Model_vmaRHTS_R2019b_2/Feedback Force Computation3 ==
  "[x_est, theta_est] (m,rad)" : Inport
  Derivative : Derivative
  Derivative1 : Derivative
  Gain1 : Gain  Gain=KPrt  Multiplication=Matrix(K*u) (u vector)
  Gain2 : Gain  Gain=CPrt  Multiplication=Matrix(K*u) (u vector)
  Gain3 : Gain  Gain=MPrt  Multiplication=Matrix(K*u) (u vector)
  Sum : Sum  Inputs=+|+|+
  Output : Outport
  wires:
  Derivative1/1 -> Gain3/1
  Gain2/1 -> Sum/2
  Derivative/1 -> Gain2/1, Derivative1/1
  Gain1/1 -> Sum/1
  Sum/1 -> Output/1
  Gain3/1 -> Sum/3
  "[x_est, theta_est] (m,rad)"/1 -> Derivative/1, Gain1/1

== system New_Model_vmaRHTS_R2019b_2/Feedback Force Guyan ==
  "[x_est, theta_est] (m,rad)" : Inport
  Derivative1 : Derivative
  Derivative2 : Derivative
  Gain1 : Gain  Gain=KPrt  Multiplication=Matrix(K*u) (u vector)
  Gain2 : Gain  Gain=CPrt  Multiplication=Matrix(K*u) (u vector)
  Gain3 : Gain  Gain=MPrt  Multiplication=Matrix(K*u) (u vector)
  Sum : Sum  Inputs=+|+|+
  Output : Outport
  wires:
  Derivative1/1 -> Gain3/1
  Gain2/1 -> Sum/2
  Derivative2/1 -> Gain2/1, Derivative1/1
  Gain1/1 -> Sum/1
  Sum/1 -> Output/1
  Gain3/1 -> Sum/3
  "[x_est, theta_est] (m,rad)"/1 -> Derivative2/1, Gain1/1

== system New_Model_vmaRHTS_R2019b_2/Feedback Force Guyan1 ==
  "[x_est, theta_est] (m,rad)" : Inport
  Derivative1 : Derivative
  Gain1 : Gain  Gain=KPrt  Multiplication=Matrix(K*u) (u vector)
  Gain2 : Gain  Gain=CPrt  Multiplication=Matrix(K*u) (u vector)
  Gain3 : Gain  Gain=MPrt  Multiplication=Matrix(K*u) (u vector)
  Sum : Sum  Inputs=+|+|+
  Output : Outport
  wires:
  Derivative1/1 -> Gain3/1
  Gain2/1 -> Sum/2
  ? -> Gain2/1, Derivative1/1
  Gain1/1 -> Sum/1
  Sum/1 -> Output/1
  Gain3/1 -> Sum/3
  "[x_est, theta_est] (m,rad)"/1 -> Gain1/1

== system New_Model_vmaRHTS_R2019b_2/ 1/Ground motion record ==
  From File : FromFile  FileName=ElCentroAccelNoScaling.mat  SampleTime=dt
  From File1 : FromFile  FileName=KobeAccelNoScaling.mat  SampleTime=dt
  From File2 : FromFile  FileName=MorganAccelNoScaling.mat  SampleTime=dt
  El Centro : Outport
  Kobe : Outport  Port=2
  Morgan : Outport  Port=3
  wires:
  From File/1 -> El Centro/1
  From File2/1 -> Morgan/1
  From File1/1 -> Kobe/1

== system New_Model_vmaRHTS_R2019b_2/ 2/Ground motion record ==
  From File : FromFile  FileName=D:\matlab\SimTool_maRTHS_BenchM_V4 R2019b\Support_files\Ground_motions\ElCentroAccelNoScaling.mat  SampleTime=dt
  From File1 : FromFile  FileName=D:\matlab\SimTool_maRTHS_BenchM_V4 R2019b\Support_files\Ground_motions\KobeAccelNoScaling.mat  SampleTime=dt
  From File2 : FromFile  FileName=D:\matlab\SimTool_maRTHS_BenchM_V4 R2019b\Support_files\Ground_motions\MorganAccelNoScaling.mat  SampleTime=dt
  El Centro : Outport
  Kobe : Outport  Port=2
  Morgan : Outport  Port=3
  wires:
  From File/1 -> El Centro/1
  From File2/1 -> Morgan/1
  From File1/1 -> Kobe/1

== system New_Model_vmaRHTS_R2019b_2/ 3/Ground motion record ==
  From File : FromFile  FileName=D:\matlab\SimTool_maRTHS_BenchM_V4 R2019b\Support_files\Ground_motions\ElCentroAccelNoScaling.mat  SampleTime=dt
  From File1 : FromFile  FileName=D:\matlab\SimTool_maRTHS_BenchM_V4 R2019b\Support_files\Ground_motions\KobeAccelNoScaling.mat  SampleTime=dt
  From File2 : FromFile  FileName=D:\matlab\SimTool_maRTHS_BenchM_V4 R2019b\Support_files\Ground_motions\MorganAccelNoScaling.mat  SampleTime=dt
  El Centro : Outport
  Kobe : Outport  Port=2
  Morgan : Outport  Port=3
  wires:
  From File/1 -> El Centro/1
  From File2/1 -> Morgan/1
  From File1/1 -> Kobe/1

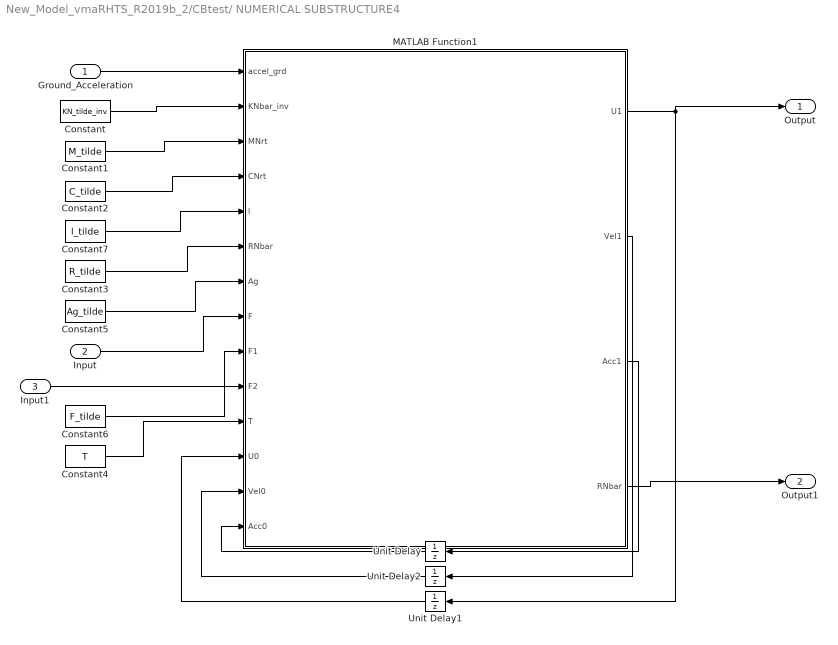
== system New_Model_vmaRHTS_R2019b_2/CBtest/ NUMERICAL SUBSTRUCTURE4 ==
  Ground_Acceleration : Inport
  Input : Inport  Port=2
  Input1 : Inport  Port=3
  Constant : Constant  Value=KN_tilde_inv  VectorParams1D=off
  Constant1 : Constant  Value=M_tilde  VectorParams1D=off
  Constant2 : Constant  Value=C_tilde  VectorParams1D=off
  Constant3 : Constant  Value=R_tilde  VectorParams1D=off
  Constant4 : Constant  Value=T  VectorParams1D=off
  Constant5 : Constant  Value=Ag_tilde  VectorParams1D=off
  Constant6 : Constant  Value=F_tilde  VectorParams1D=off
  Constant7 : Constant  Value=l_tilde  VectorParams1D=off
  MATLAB Function1 : MATLAB Function  TreatAsAtomicUnit=on
  Unit Delay : UnitDelay  SampleTime=-1  HasFrameUpgradeWarning=on
  Unit Delay1 : UnitDelay  SampleTime=-1  HasFrameUpgradeWarning=on
  Unit Delay2 : UnitDelay  SampleTime=-1  HasFrameUpgradeWarning=on
  Output : Outport
  Output1 : Outport  Port=2
  wires:
  Ground_Acceleration/1 -> MATLAB Function1/1(accel_grd)
  Constant/1 -> MATLAB Function1/2(KNbar_inv)
  Constant1/1 -> MATLAB Function1/3(MNrt)
  Constant2/1 -> MATLAB Function1/4(CNrt)
  Constant7/1 -> MATLAB Function1/5(l)
  Unit Delay2/1 -> MATLAB Function1/13(Vel0)
  Unit Delay/1 -> MATLAB Function1/14(Acc0)
  MATLAB Function1/2(Vel1) -> Unit Delay2/1
  MATLAB Function1/3(Acc1) -> Unit Delay/1
  Constant5/1 -> MATLAB Function1/7(Ag)
  Unit Delay1/1 -> MATLAB Function1/12(U0)
  Constant3/1 -> MATLAB Function1/6("RNbar ")
  Input/1 -> MATLAB Function1/8(F)
  MATLAB Function1/1(U1) -> Output/1, Unit Delay1/1
  Constant6/1 -> MATLAB Function1/9(F1)
  MATLAB Function1/4(RNbar) -> Output1/1
  Input1/1 -> MATLAB Function1/10(F2)
  Constant4/1 -> MATLAB Function1/11(T)

== system New_Model_vmaRHTS_R2019b_2/CBtest/Feedback Force Computation4 ==
  "[x_est, theta_est] (m,rad)" : Inport
  Derivative : Derivative
  Derivative1 : Derivative
  Gain1 : Gain  Gain=Kp_tilde  Multiplication=Matrix(K*u) (u vector)
  Gain2 : Gain  Gain=Cp_tilde  Multiplication=Matrix(K*u) (u vector)
  Gain3 : Gain  Gain=Mp_tilde  Multiplication=Matrix(K*u) (u vector)
  Sum : Sum  Inputs=+|+|+
  Output : Outport
  wires:
  Derivative1/1 -> Gain3/1
  Gain2/1 -> Sum/2
  Derivative/1 -> Gain2/1, Derivative1/1
  Gain1/1 -> Sum/1
  Sum/1 -> Output/1
  Gain3/1 -> Sum/3
  "[x_est, theta_est] (m,rad)"/1 -> Derivative/1, Gain1/1

== matlab function New_Model_vmaRHTS_R2019b_2/ Ps SUBSTRUCTURE1/MATLAB Function1 ==
  data: U1 output; Vel1 output; Acc1 output; accel_grd input; KNbar_inv input; MNrt input; CNrt input; l input; RNbar input; Ag input; F3 input; F78 input; locate3 input; U0 input; Vel0 input; Acc0 input; a0 parameter; a1 parameter; a2 parameter; a3 parameter; a4 parameter; a5 parameter; a6 parameter; a7 parameter; RNbar output
function [U1,Vel1,Acc1,RNbar]=fcn2(accel_grd,KNbar_inv, MNrt, CNrt,l,RNbar,Ag,F3,F78,locate3,...
    U0,Vel0,Acc0, a0, a1, a2, a3, a4, a5, a6, a7)
             
    % 该求解方法为 Newmark-β法        
    % ============================
	% *  Update next iteration   *
	% ============================
    ndof = length(KNbar_inv);
    U1   = zeros(ndof,1);
    Vel1 = zeros(ndof,1);
    Acc1 = zeros(ndof,1);
    F = zeros(6,1);
    F(3,1) = F3;
    F(5:6,1) = F78;
    % ============================
	% *  Feedback Force / Moment *
	% ============================
%     F(27) = -FB_force;
%     F(14) = -FB_moment;

    % ==========================
	% *     Update Matrices    *
	% ==========================
    Ag  = accel_grd * l;
   	% ==========================
	% * 	  Form Rbar  	   *
	% ==========================
	RNbar = ( (MNrt * ((a0*U0)+(a2*Vel0)+(a3*Acc0))) + ...
		     (CNrt * ((a1*U0)+(a4*Vel0)+(a5*Acc0))) -F-  (MNrt * Ag) );
    % ==========================
	% * Solve for Displacement *
	% ==========================
	U1 = KNbar_inv * RNbar;
    
	% ============================
	% * Compute Velocity & Accel *
	% ============================
	Acc1=a0*(U1-U0)-a2*Vel0-a3*Acc0;
	Vel1=Vel0+a7*Acc1+a6*Acc0;

end

== matlab function New_Model_vmaRHTS_R2019b_2/ NUMERICAL SUBSTRUCTURE1/MATLAB Function1 ==
  data: U1 output; Vel1 output; Acc1 output; accel_grd input; KNbar_inv input; MNrt input; CNrt input; l input; RNbar input; Ag input; F input; F1 input; F2 input; locate2 input; U0 input; Vel0 input; Acc0 input; a0 parameter; a1 parameter; a2 parameter; a3 parameter; a4 parameter; a5 parameter; a6 parameter; a7 parameter; RNbar output
function [U1,Vel1,Acc1,RNbar]=fcn2(accel_grd,KNbar_inv, MNrt, CNrt,l,RNbar,Ag,F,F1,F2,locate2,...
    U0,Vel0,Acc0, a0, a1, a2, a3, a4, a5, a6, a7)
             
    % 该求解方法为 Newmark-β法        
    % ============================
	% *  Update next iteration   *
	% ============================
    ndof = length(KNbar_inv);
    U1   = zeros(ndof,1);
    Vel1 = zeros(ndof,1);
    Acc1 = zeros(ndof,1);
    
    F1(locate2) = F;
    % ============================
	% *  Feedback Force / Moment *
	% ============================
%     F(27) = -FB_force;
%     F(14) = -FB_moment;

    % ==========================
	% *     Update Matrices    *
	% ==========================
    Ag  = accel_grd * l;
   	% ==========================
	% * 	  Form Rbar  	   *
	% ==========================
	%RNbar = ( (MNrt * ((a0*U0)+(a2*Vel0)+(a3*Acc0))) + ...
	%	     (CNrt * ((a1*U0)+(a4*Vel0)+(a5*Acc0))) -F1-  (MNrt * Ag) );

    RNbar = ( (MNrt * ((a0*U0)+(a2*Vel0)+(a3*Acc0))) + ...
		     (CNrt * ((a1*U0)+(a4*Vel0)+(a5*Acc0))) -F1-  (MNrt * Ag) );
    
    % ==========================
	% * Solve for Displacement *
	% ==========================
	U1 = KNbar_inv * RNbar;
    
	% ============================
	% * Compute Velocity & Accel *
	% ============================
	Acc1=a0*(U1-U0)-a2*Vel0-a3*Acc0;
	Vel1=Vel0+a7*Acc1+a6*Acc0;

end

== matlab function New_Model_vmaRHTS_R2019b_2/ REFERENCE STRUCTURE/MATLAB Function1 ==
  data: U1 output; Vel1 output; Acc1 output; accel_grd input; Kbar_inv input; MNrt input; CNrt input; l input; Rbar input; Ag input; U0 input; Vel0 input; Acc0 input; a0 parameter; a1 parameter; a2 parameter; a3 parameter; a4 parameter; a5 parameter; a6 parameter; a7 parameter; Rbar output
function [U1,Vel1,Acc1,Rbar]=fcn1(accel_grd,Kbar_inv, MNrt, CNrt,l,Rbar,Ag,...
    U0,Vel0,Acc0, a0, a1, a2, a3, a4, a5, a6, a7)
             
             
    % ============================
	% *  Update next iteration   *
	% ============================
    ndof = length(Kbar_inv);
    U1   = zeros(ndof,1);
    Vel1 = zeros(ndof,1);
    Acc1 = zeros(ndof,1);
    
    % ============================
	% *  Feedback Force / Moment *
	% ============================
%     F(27) = -FB_force;
%     F(14) = -FB_moment;

    % ==========================
	% *     Update Matrices    *
	% ==========================
    Ag  = accel_grd * l;
    
   	% ==========================
	% * 	  Form Rbar  	   *
	% ==========================
	Rbar = ( (MNrt * ((a0*U0)+(a2*Vel0)+(a3*Acc0))) + ...
		     (CNrt * ((a1*U0)+(a4*Vel0)+(a5*Acc0))) -  (MNrt * Ag) );
    % ==========================
	% * Solve for Displacement *
	% ==========================
	U1 = Kbar_inv * Rbar;
    
	% ============================
	% * Compute Velocity & Accel *
	% ============================
	Acc1=a0*(U1-U0)-a2*Vel0-a3*Acc0;
	Vel1=Vel0+a7*Acc1+a6*Acc0;

end

== matlab function New_Model_vmaRHTS_R2019b_2/ NUMERICAL SUBSTRUCTURE/MATLAB Function1 ==
  data: U1 output; Vel1 output; Acc1 output; accel_grd input; KNbar_inv input; MNrt input; CNrt input; l input; RNbar input; Ag input; F1 input; F2 input; locate3 input; U0 input; Vel0 input; Acc0 input; a0 parameter; a1 parameter; a2 parameter; a3 parameter; a4 parameter; a5 parameter; a6 parameter; a7 parameter; RNbar output
function [U1,Vel1,Acc1,RNbar]=fcn2(accel_grd,KNbar_inv, MNrt, CNrt,l,RNbar,Ag,F1,F2,locate3,...
    U0,Vel0,Acc0, a0, a1, a2, a3, a4, a5, a6, a7)
             
    % 该求解方法为 Newmark-β法        
    % ============================
	% *  Update next iteration   *
	% ============================
    ndof = length(KNbar_inv);
    U1   = zeros(ndof,1);
    Vel1 = zeros(ndof,1);
    Acc1 = zeros(ndof,1);
    F = zeros(11,1);
    F(2,1) = F1;
    F(5:9) = F2;
    % ============================
	% *  Feedback Force / Moment *
	% ============================
%     F(27) = -FB_force;
%     F(14) = -FB_moment;

    % ==========================
	% *     Update Matrices    *
	% ==========================
    Ag  = accel_grd * l;
   	% ==========================
	% * 	  Form Rbar  	   *
	% ==========================
	RNbar = ( (MNrt * ((a0*U0)+(a2*Vel0)+(a3*Acc0))) + ...
		     (CNrt * ((a1*U0)+(a4*Vel0)+(a5*Acc0))) -F-  (MNrt * Ag) );
    % ==========================
	% * Solve for Displacement *
	% ==========================
	U1 = KNbar_inv * RNbar;
    
	% ============================
	% * Compute Velocity & Accel *
	% ============================
	Acc1=a0*(U1-U0)-a2*Vel0-a3*Acc0;
	Vel1=Vel0+a7*Acc1+a6*Acc0;

end

== matlab function New_Model_vmaRHTS_R2019b_2/ NUMERICAL Guyan/MATLAB Function1 ==
  data: U1 output; Vel1 output; Acc1 output; accel_grd input; KNbar_inv input; MNrt input; CNrt input; l input; RNbar input; Ag input; F input; F1 input; locate2 input; U0 input; Vel0 input; Acc0 input; a0 parameter; a1 parameter; a2 parameter; a3 parameter; a4 parameter; a5 parameter; a6 parameter; a7 parameter; RNbar output
function [U1,Vel1,Acc1,RNbar]=fcn2(accel_grd,KNbar_inv, MNrt, CNrt,l,RNbar,Ag,F,F1,locate2,...
    U0,Vel0,Acc0, a0, a1, a2, a3, a4, a5, a6, a7)
             
    % 该求解方法为 Newmark-β法        
    % ============================
	% *  Update next iteration   *
	% ============================
    ndof = length(KNbar_inv);
    U1   = zeros(ndof,1);
    Vel1 = zeros(ndof,1);
    Acc1 = zeros(ndof,1);
    
    F1(locate2) = F;
    % ============================
	% *  Feedback Force / Moment *
	% ============================
%     F(27) = -FB_force;
%     F(14) = -FB_moment;

    % ==========================
	% *     Update Matrices    *
	% ==========================
    Ag  = accel_grd * l;
   	% ==========================
	% * 	  Form Rbar  	   *
	% ==========================
	%RNbar = ( (MNrt * ((a0*U0)+(a2*Vel0)+(a3*Acc0))) + ...
	%	     (CNrt * ((a1*U0)+(a4*Vel0)+(a5*Acc0))) -F1-  (MNrt * Ag) );

    RNbar = ( (MNrt * ((a0*U0)+(a2*Vel0)+(a3*Acc0))) + ...
		     (CNrt * ((a1*U0)+(a4*Vel0)+(a5*Acc0))) -F1-  (MNrt * Ag) );
    
    % ==========================
	% * Solve for Displacement *
	% ==========================
	U1 = KNbar_inv * RNbar;
    
	% ============================
	% * Compute Velocity & Accel *
	% ============================
	Acc1=a0*(U1-U0)-a2*Vel0-a3*Acc0;
	Vel1=Vel0+a7*Acc1+a6*Acc0;

end

== matlab function New_Model_vmaRHTS_R2019b_2/ NUMERICAL Guyan1/MATLAB Function1 ==
  data: U1 output; Vel1 output; Acc1 output; accel_grd input; KNbar_inv input; MNrt input; CNrt input; l input; RNbar input; Ag input; F input; F1 input; locate2 input; U0 input; Vel0 input; Acc0 input; a0 parameter; a1 parameter; a2 parameter; a3 parameter; a4 parameter; a5 parameter; a6 parameter; a7 parameter; RNbar output
function [U1,Vel1,Acc1,RNbar]=fcn2(accel_grd,KNbar_inv, MNrt, CNrt,l,RNbar,Ag,F,F1,locate2,...
    U0,Vel0,Acc0, a0, a1, a2, a3, a4, a5, a6, a7)
             
    % 该求解方法为 Newmark-β法        
    % ============================
	% *  Update next iteration   *
	% ============================
    ndof = length(KNbar_inv);
    U1   = zeros(ndof,1);
    Vel1 = zeros(ndof,1);
    Acc1 = zeros(ndof,1);
    
    F1(locate2) = F;
    % ============================
	% *  Feedback Force / Moment *
	% ============================
%     F(27) = -FB_force;
%     F(14) = -FB_moment;

    % ==========================
	% *     Update Matrices    *
	% ==========================
    Ag  = accel_grd * l;
   	% ==========================
	% * 	  Form Rbar  	   *
	% ==========================
	%RNbar = ( (MNrt * ((a0*U0)+(a2*Vel0)+(a3*Acc0))) + ...
	%	     (CNrt * ((a1*U0)+(a4*Vel0)+(a5*Acc0))) -F1-  (MNrt * Ag) );

    RNbar = ( (MNrt * ((a0*U0)+(a2*Vel0)+(a3*Acc0))) + ...
		     (CNrt * ((a1*U0)+(a4*Vel0)+(a5*Acc0))) -F1-  (MNrt * Ag) );
    
    % ==========================
	% * Solve for Displacement *
	% ==========================
	U1 = KNbar_inv * RNbar;
    
	% ============================
	% * Compute Velocity & Accel *
	% ============================
	Acc1=a0*(U1-U0)-a2*Vel0-a3*Acc0;
	Vel1=Vel0+a7*Acc1+a6*Acc0;

end

== matlab function New_Model_vmaRHTS_R2019b_2/ NUMERICAL SUBSTRUCTURE2/MATLAB Function1 ==
  data: U1 output; Vel1 output; Acc1 output; accel_grd input; KNbar_inv input; MNrt input; CNrt input; l input; RNbar input; Ag input; F input; F1 input; F2 input; locate2 input; U0 input; Vel0 input; Acc0 input; a0 parameter; a1 parameter; a2 parameter; a3 parameter; a4 parameter; a5 parameter; a6 parameter; a7 parameter; RNbar output
function [U1,Vel1,Acc1,RNbar]=fcn2(accel_grd,KNbar_inv, MNrt, CNrt,l,RNbar,Ag,F,F1,F2,locate2,...
    U0,Vel0,Acc0, a0, a1, a2, a3, a4, a5, a6, a7)
             
    % 该求解方法为 Newmark-β法        
    % ============================
	% *  Update next iteration   *
	% ============================
    ndof = length(KNbar_inv);
    U1   = zeros(ndof,1);
    Vel1 = zeros(ndof,1);
    Acc1 = zeros(ndof,1);
    
    F1 = F;
    % ============================
	% *  Feedback Force / Moment *
	% ============================
%     F(27) = -FB_force;
%     F(14) = -FB_moment;

    % ==========================
	% *     Update Matrices    *
	% ==========================
    Ag  = accel_grd * l;
   	% ==========================
	% * 	  Form Rbar  	   *
	% ==========================
	%RNbar = ( (MNrt * ((a0*U0)+(a2*Vel0)+(a3*Acc0))) + ...
	%	     (CNrt * ((a1*U0)+(a4*Vel0)+(a5*Acc0))) -F1-  (MNrt * Ag) );

    RNbar = ( (MNrt * ((a0*U0)+(a2*Vel0)+(a3*Acc0))) + ...
		     (CNrt * ((a1*U0)+(a4*Vel0)+(a5*Acc0))) -F1-  (MNrt * Ag) );
    
    % ==========================
	% * Solve for Displacement *
	% ==========================
	U1 = KNbar_inv * RNbar;
    
	% ============================
	% * Compute Velocity & Accel *
	% ============================
	Acc1=a0*(U1-U0)-a2*Vel0-a3*Acc0;
	Vel1=Vel0+a7*Acc1+a6*Acc0;

end

== matlab function New_Model_vmaRHTS_R2019b_2/ NUMERICAL SUBSTRUCTURE3/MATLAB Function1 ==
  data: U1 output; Vel1 output; Acc1 output; accel_grd input; KNbar_inv input; MNrt input; CNrt input; l input; RNbar input; Ag input; F input; F1 input; F2 input; T input; U0 input; Vel0 input; Acc0 input; a0 parameter; a1 parameter; a2 parameter; a3 parameter; a4 parameter; a5 parameter; a6 parameter; a7 parameter; RNbar output
function [U1,Vel1,Acc1,RNbar]=fcn2(accel_grd,KNbar_inv, MNrt, CNrt,l,RNbar,Ag,F,F1,F2,T,...
    U0,Vel0,Acc0, a0, a1, a2, a3, a4, a5, a6, a7)
             
    % 该求解方法为 Newmark-β法        
    % ============================
	% *  Update next iteration   *
	% ============================
    ndof = length(KNbar_inv);
    U1   = zeros(ndof,1);
    Vel1 = zeros(ndof,1);
    Acc1 = zeros(ndof,1);
    
    F1 = F;
    % ============================
	% *  Feedback Force / Moment *
	% ============================
%     F(27) = -FB_force;
%     F(14) = -FB_moment;

    % ==========================
	% *     Update Matrices    *
	% ==========================
    Ag  = accel_grd * l;
   	% ==========================
	% * 	  Form Rbar  	   *
	% ==========================
	%RNbar = ( (MNrt * ((a0*U0)+(a2*Vel0)+(a3*Acc0))) + ...
	%	     (CNrt * ((a1*U0)+(a4*Vel0)+(a5*Acc0))) -F1-  (MNrt * Ag) );

    RNbar = ( (MNrt * ((a0*U0)+(a2*Vel0)+(a3*Acc0))) + ...
		     (CNrt * ((a1*U0)+(a4*Vel0)+(a5*Acc0))) -F1-  (MNrt * Ag) );
    
    % ==========================
	% * Solve for Displacement *
	% ==========================
	U1 = KNbar_inv * RNbar;
    
	% ============================
	% * Compute Velocity & Accel *
	% ============================
	Acc1=a0*(U1-U0)-a2*Vel0-a3*Acc0;
	Vel1=Vel0+a7*Acc1+a6*Acc0;

end
